simulink model "LongitudinalControlDesign"  (R2020b)
settings: Solver=ode15s  StartTime=0.0  StopTime=500  RelTol=1e-3
values from neighbouring files (symbols this model uses):
  actuatorDen = [1,   actuatorTimeConstant]    [LateralControl.m]    (also in LongitudinalControl.m)
  actuatorNum = actuatorGain*actuatorTimeConstant    (= 5)    [LateralControl.m]    (also in LongitudinalControl.m)
  ALong = [	-0.0141295      0.0580298       0           -9.81 ... (first row only)    [LongitudinalControl.m]
  BLong = [	-0.1703679 ... (first row only)    [LongitudinalControl.m]
  CLong = [1,     0,  0,  0 ... (first row only)    [LongitudinalControl.m]
  DGain = PGain*Td    (= 0.156)    [LateralControl.m]    (also in LongitudinalControl.m = 0.0211)
  DLong = [0 ... (first row only)    [LongitudinalControl.m]
  InitialConditions = [0 ... (first row only)    [LateralControl.m]    (also in LongitudinalControl.m)
  PGain = 1.56    [LateralControl.m]    (also in LongitudinalControl.m = 0.211)
  stepCommand = 0    [LateralControl.m]    (also in LongitudinalControl.m = 1)
libraries: slpidlib x1
settings Model: Creator=Antonis Kantounias  LastModifiedBy=Antonis Kantounias

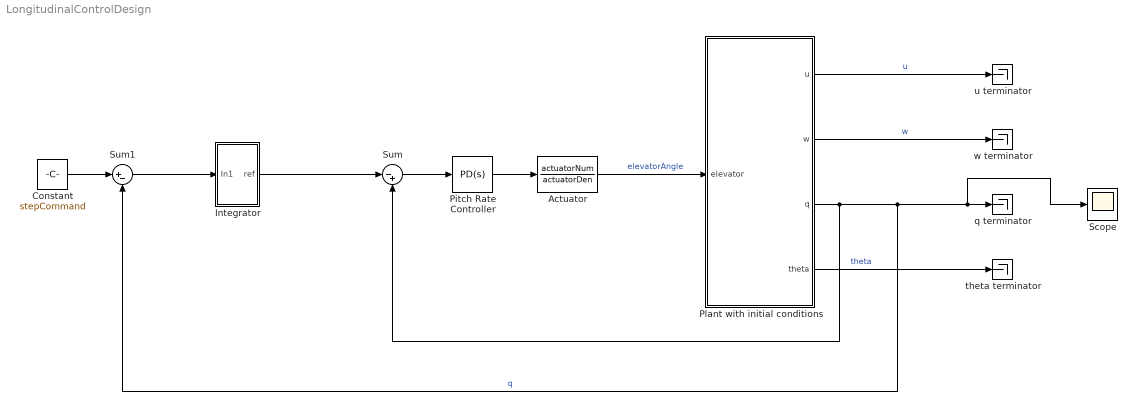
== system LongitudinalControlDesign ==
  Actuator : TransferFcn  Numerator=actuatorNum  Denominator=actuatorDen
  Constant : Constant  Value=stepCommand
  Integrator : Subsystem
  Pitch Rate Controller : slpidlib/PID Controller  Controller=PD  Form=Parallel  TimeDomain=Continuous-time  UseExternalTs=off  SampleTime=-1  IntegratorMethod=Forward Euler  FilterMethod=Forward Euler  ControllerParametersSource=internal  P=PGain  I=1  D=DGain  UseFilter=on  N=100  TunerSelectOption=Transfer Function Based (PID Tuner App)  InitialConditionSource=internal  InitialConditionForIntegrator=0  InitialConditionForFilter=0  DifferentiatorICPrevScaledInput=0  ExternalReset=none  TrackingMode=off  Kt=1  LimitOutput=off  SatLimitsSource=internal  UpperSaturationLimit=inf  LowerSaturationLimit=-inf  LinearizeAsGain=on  AntiWindupMode=none  Kb=1  POutMin=[]  POutMax=[]  IOutMin=[]  IOutMax=[]  DOutMin=[]  DOutMax=[]  NOutMin=[]  NOutMax=[]  SumOutMin=[]  SumOutMax=[]  SaturationOutMin=[]  SaturationOutMax=[]  PParamMin=[]  PParamMax=[]  IParamMin=[]  IParamMax=[]  DParamMin=[]  DParamMax=[]  NParamMin=[]  NParamMax=[]  KbParamMin=[]  KbParamMax=[]  KtParamMin=[]  KtParamMax=[]  KbOutMin=[]  KbOutMax=[]  KtOutMin=[]  KtOutMax=[]  IntegratorOutMin=[]  IntegratorOutMax=[]  FilterOutMin=[]  FilterOutMax=[]  SumI1OutMin=[]  SumI1OutMax=[]  SumI2OutMin=[]  SumI2OutMax=[]  SumI3OutMin=[]  SumI3OutMax=[]  SumI4OutMin=[]  SumI4OutMax=[]  SumDOutMin=[]  SumDOutMax=[]  DifferentiatorOutMin=[]  DifferentiatorOutMax=[]  FilterDiffOutCoefMin=[]  FilterDiffOutCoefMax=[]  ReciprocalOutMin=[]  ReciprocalOutMax=[]  SumDenOutMin=[]  SumDenOutMax=[]  SumNumOutMin=[]  SumNumOutMax=[]  DivideOutMin=[]  DivideOutMax=[]  UdiffTsProdOutMin=[]  UdiffTsProdOutMax=[]  NTsProdOutMin=[]  NTsProdOutMax=[]  UintegralTsProdOutMin=[]  UintegralTsProdOutMax=[]  UngainTsProdOutMin=[]  UngainTsProdOutMax=[]  IntegratorContinuousStateAttributes=''  IntegratorStateMustResolveToSignalObject=off  IntegratorRTWStateStorageClass=Auto  FilterContinuousStateAttributes=''  FilterStateMustResolveToSignalObject=off  FilterRTWStateStorageClass=Auto  ParallelPVariant=InternalParameters  IdealPVariant=Disabled  IVariant=Disabled  DVariant=InternalParameters  IntegratorVariant=Disabled  SatVariant=Disabled  AWVariant=Disabled  PCopyVariant=Disabled  TRVariant=Disabled  FdbkBlocksVariant=Forward  IdealPFdbkVariant=Disabled  SatFdbkVariant=Disabled  DerivativeFilterVariant=ContFilter  NVariant=InternalParameters  NCopyVariant=Disabled  FilterICVariant=InternalICsFilter  IntegratorICVariant=Disabled  ExternalResetVariant=Disabled  TRSumVariant=Passthrough  SumFdbkVariant=Disabled  SumVariant=Sum_PD  TsampFilterVariant=InternalTs  TsampNgainVariant=Passthrough  TsampIntegralVariant=Disabled_SignalSpec  ExternalSaturationOutDataTypeStr=Inherit: Same as second input
  Plant with initial conditions : Subsystem
  Scope : Scope
  Sum : Sum  Inputs=|-+
  Sum1 : Sum  Inputs=|+-
  q terminator : Terminator
  theta terminator : Terminator
  u terminator : Terminator
  w terminator : Terminator
  wires:
  Plant with initial conditions/3(q) -> Sum/2, Scope/1, q terminator/1, Sum1/2  "q"
  Plant with initial conditions/1(u) -> u terminator/1  "u"
  Plant with initial conditions/2(w) -> w terminator/1  "w"
  Plant with initial conditions/4(theta) -> theta terminator/1  "theta"
  Sum/1 -> Pitch Rate Controller/1
  Pitch Rate Controller/1 -> Actuator/1
  Actuator/1 -> Plant with initial conditions/1(elevator)  "elevatorAngle"
  Constant/1 -> Sum1/1
  Sum1/1 -> Integrator/1(In1)
  Integrator/1(ref) -> Sum/1

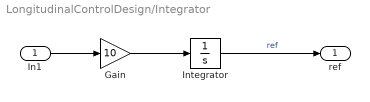
== system LongitudinalControlDesign/Integrator ==
  In1 : Inport
  Gain : Gain  Gain=10
  Integrator : Integrator
  ref : Outport
  wires:
  In1/1 -> Gain/1
  Gain/1 -> Integrator/1
  Integrator/1 -> ref/1  "ref"

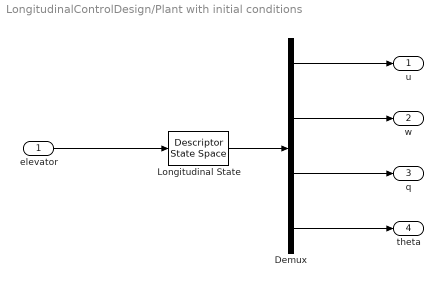
== system LongitudinalControlDesign/Plant with initial conditions ==
  elevator : Inport
  Demux : Demux
  "Longitudinal State " : DescriptorStateSpace  E=ELong  A=ALong  B=BLong  C=CLong  D=DLong  InitialCondition=InitialConditions  ContinuousStateAttributes='LongitudinalSystem'
  u : Outport
  w : Outport  Port=2
  q : Outport  Port=3
  theta : Outport  Port=4
  wires:
  "Longitudinal State "/1 -> Demux/1
  Demux/4 -> theta/1
  Demux/1 -> u/1
  Demux/3 -> q/1
  Demux/2 -> w/1
  elevator/1 -> "Longitudinal State "/1
